simulink model "WholeAssembly"  (R2019a)
settings: Solver=VariableStepAuto  StartTime=0.0  StopTime=160  RelTol=1e-3
values from neighbouring files (symbols this model uses):
  d = 0.01    [workspace.mat]
  IR = [10 10.0005046937 10.0010093873 10.001514081 10.0020187746 10.0025234683 10.0030281619 10.0035328556 10.0040375492 10.0045422429 10.0050469365 10.0055516302 ... (9908 elements, 9908x1)]    [workspace.mat]
  Q = 31.2    [workspace.mat]
  T = [0 0.00605632381145 0.0121126476229 0.0181689714343 0.0242252952458 0.0302816190572 0.0363379428687 0.0423942666801 0.0484505904916 0.054506914303 0.0605632381145 0.0666195619259 ... (9908 elements, 9908x1)]    [workspace.mat]
undefined symbols (not defined in the file or in its folder): ocv, soc
libraries: simulink x3
settings Model: Creator=sujan  LastModifiedBy=sujan

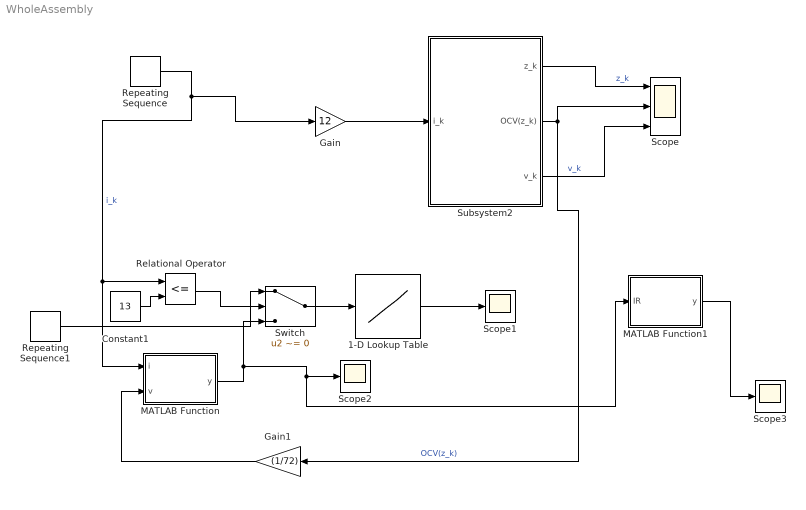
== system WholeAssembly ==
  1-D Lookup Table : Lookup_n-D  NumberOfTableDimensions=1  BreakpointsForDimension1=T  Table=IR  InternalRulePriority=Speed  RndMeth=Simplest  InputSameDT=on
  Constant1 : Constant  Value=13
  Gain : Gain  Gain=12
  Gain1 : Gain  Gain=(1/72)
  MATLAB Function : MATLAB Function  TreatAsAtomicUnit=on
  MATLAB Function1 : MATLAB Function  TreatAsAtomicUnit=on
  Relational Operator : RelationalOperator  Operator=<=  OutDataTypeStr=boolean  RndMeth=Simplest
  Repeating Sequence : simulink/Sources/Repeating Sequence  rep_seq_t=time  rep_seq_y=I
  Repeating Sequence1 : simulink/Sources/Repeating Sequence  rep_seq_t=t  rep_seq_y=T
  Scope : Scope  NumInputPorts=3
  Scope1 : Scope
  Scope2 : Scope
  Scope3 : Scope
  Subsystem2 : Subsystem
  Switch : Switch  Criteria=u2 ~= 0
  wires:
  Subsystem2/2(OCV(z_k)) -> Scope/2, Gain1/1  "OCV(z_k)"
  Subsystem2/3(v_k) -> Scope/3  "v_k"
  Repeating Sequence/1 -> MATLAB Function/1(i), Relational Operator/1, Gain/1  "i_k"
  Subsystem2/1(z_k) -> Scope/1  "z_k"
  Gain/1 -> Subsystem2/1(i_k)
  1-D Lookup Table/1 -> Scope1/1
  Switch/1 -> 1-D Lookup Table/1
  Repeating Sequence1/1 -> Switch/1
  Relational Operator/1 -> Switch/2
  Constant1/1 -> Relational Operator/2
  MATLAB Function/1(y) -> MATLAB Function1/1(IR), Scope2/1, Switch/3
  Gain1/1 -> MATLAB Function/2(v)
  MATLAB Function1/1(y) -> Scope3/1

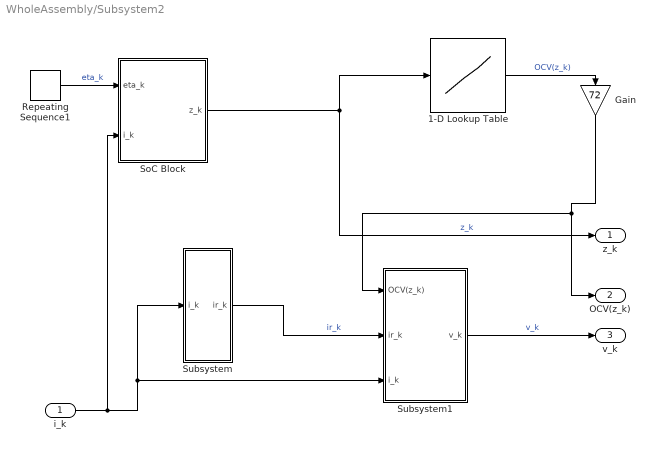
== system WholeAssembly/Subsystem2 ==
  i_k : Inport
  1-D Lookup Table : Lookup_n-D  NumberOfTableDimensions=1  LookupTableObject=Em  BreakpointsForDimension1=soc.soc  Table=ocv.ocv  InternalRulePriority=Speed  RndMeth=Simplest  InputSameDT=on
  Gain : Gain  Gain=72
  Repeating Sequence1 : simulink/Sources/Repeating Sequence  rep_seq_t=time  rep_seq_y=eta1
  "SoC Block " : Subsystem
  Subsystem : Subsystem
  Subsystem1 : Subsystem
  z_k : Outport
  OCV(z_k) : Outport  Port=2
  v_k : Outport  Port=3
  wires:
  1-D Lookup Table/1 -> Gain/1  "OCV(z_k)"
  i_k/1 -> "SoC Block "/2(i_k), Subsystem/1(i_k), Subsystem1/3(i_k)
  Subsystem1/1(v_k) -> v_k/1  "v_k"
  "SoC Block "/1(z_k) -> 1-D Lookup Table/1, z_k/1  "z_k"
  Subsystem/1(ir_k) -> Subsystem1/2(ir_k)  "ir_k"
  Repeating Sequence1/1 -> "SoC Block "/1(eta_k)  "eta_k"
  Gain/1 -> Subsystem1/1(OCV(z_k)), OCV(z_k)/1

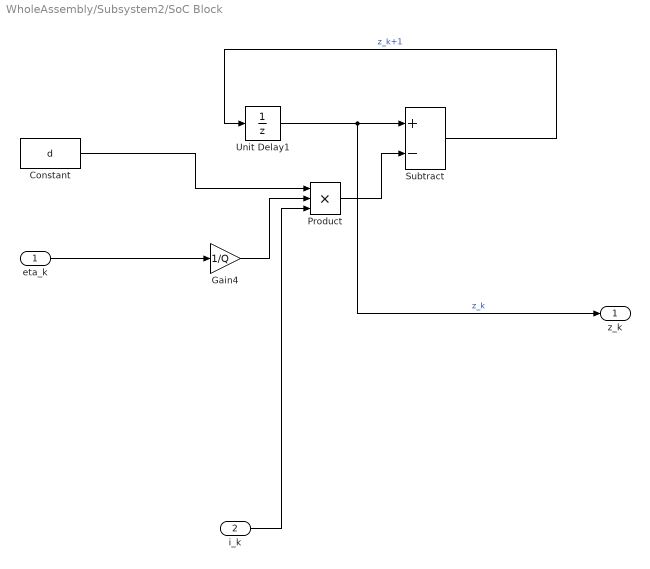
== system WholeAssembly/Subsystem2/SoC Block  ==
  eta_k : Inport
  i_k : Inport  Port=2
  Constant : Constant  Value=d
  Gain4 : Gain  Gain=1/Q
  Product : Product  Inputs=3
  Subtract : Sum  Inputs=+-
  Unit Delay1 : UnitDelay  InitialCondition=100  HasFrameUpgradeWarning=on
  z_k : Outport
  wires:
  Product/1 -> Subtract/2
  Constant/1 -> Product/1
  Unit Delay1/1 -> z_k/1, Subtract/1  "z_k"
  eta_k/1 -> Gain4/1
  Gain4/1 -> Product/2
  i_k/1 -> Product/3
  Subtract/1 -> Unit Delay1/1  "z_k+1"

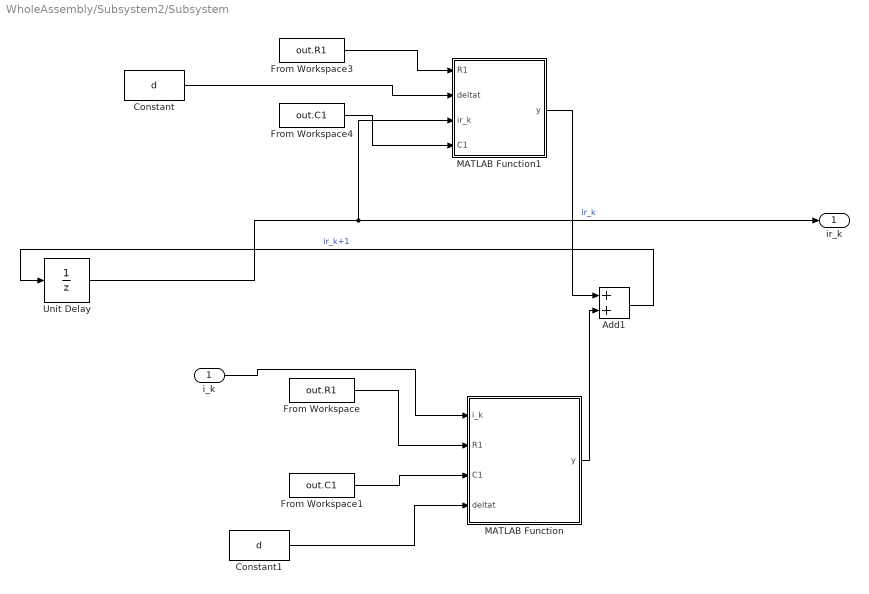
== system WholeAssembly/Subsystem2/Subsystem ==
  i_k : Inport
  Add1 : Sum
  Constant : Constant  Value=d
  Constant1 : Constant  Value=d
  From Workspace : FromWorkspace  VariableName=out.R1  SampleTime=0
  From Workspace1 : FromWorkspace  VariableName=out.C1  SampleTime=0
  From Workspace3 : FromWorkspace  VariableName=out.R1  SampleTime=0
  From Workspace4 : FromWorkspace  VariableName=out.C1  SampleTime=0
  MATLAB Function : MATLAB Function  TreatAsAtomicUnit=on
  MATLAB Function1 : MATLAB Function  TreatAsAtomicUnit=on
  Unit Delay : UnitDelay  HasFrameUpgradeWarning=on
  ir_k : Outport
  wires:
  MATLAB Function1/1(y) -> Add1/1
  Unit Delay/1 -> MATLAB Function1/3(ir_k), ir_k/1  "ir_k"
  Add1/1 -> Unit Delay/1  "ir_k+1"
  i_k/1 -> MATLAB Function/1(i_k)
  MATLAB Function/1(y) -> Add1/2
  From Workspace/1 -> MATLAB Function/2(R1)
  From Workspace4/1 -> MATLAB Function1/4(C1)
  From Workspace3/1 -> MATLAB Function1/1(R1)
  From Workspace1/1 -> MATLAB Function/3(C1)
  Constant/1 -> MATLAB Function1/2(deltat)
  Constant1/1 -> MATLAB Function/4(deltat)

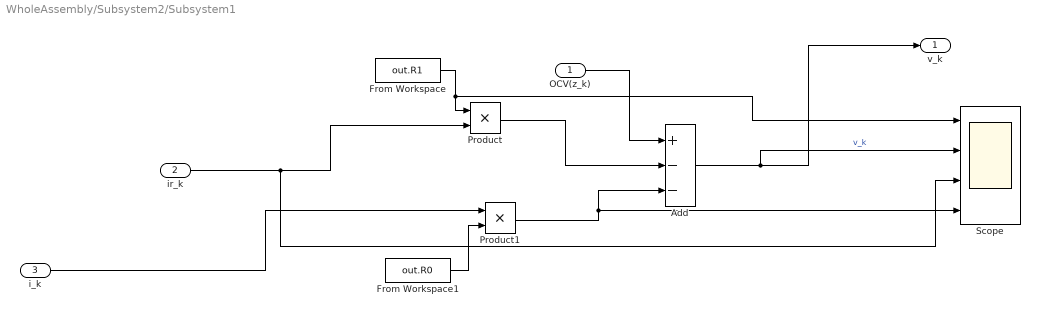
== system WholeAssembly/Subsystem2/Subsystem1 ==
  OCV(z_k) : Inport
  ir_k : Inport  Port=2
  i_k : Inport  Port=3
  Add : Sum  Inputs=+--
  From Workspace : FromWorkspace  VariableName=out.R1  SampleTime=0
  From Workspace1 : FromWorkspace  VariableName=out.R0  SampleTime=0
  Product : Product
  Product1 : Product
  Scope : Scope  NumInputPorts=4
  v_k : Outport
  wires:
  ir_k/1 -> Scope/3, Product/2
  Product/1 -> Add/2
  Product1/1 -> Scope/4, Add/3
  i_k/1 -> Product1/1
  OCV(z_k)/1 -> Add/1
  Add/1 -> Scope/2, v_k/1  "v_k"
  From Workspace1/1 -> Product1/2
  From Workspace/1 -> Scope/1, Product/1

== matlab function WholeAssembly/Subsystem2/Subsystem/MATLAB Function1 ==
  data: R1 input; deltat input; ir_k input; C1 input; y output
function y = fcn(R1,deltat, ir_k, C1)

y =ir_k*(exp(-deltat/(R1*C1)));

== matlab function WholeAssembly/Subsystem2/Subsystem/MATLAB Function ==
  data: i_k input; R1 input; C1 input; y output; deltat input
function y = fcn(i_k, R1,C1, deltat)

y = i_k*(1-exp(-deltat/(R1*C1)));

== matlab function WholeAssembly/MATLAB Function ==
  data: i input; y output; v input
function y = fcn(i,v )

y = (v/i);

== matlab function WholeAssembly/MATLAB Function1 ==
  data: IR input; y output
function y = fcn(IR)

y = ((0.36-IR)/(0.36-0.30))*100;
